simulink model "prob1"  (R2020b)
settings: Solver=VariableStepAuto  StartTime=0.0  StopTime=50.0  RelTol=1e-3
model workspace (MAT data in the model file):
  K1 = Simulink.Parameter
  K1.Value = 3
  K1.DataType = 'auto'
  K1.Dimensions = [1 1]
  K12 = Simulink.Parameter
  K12.Value = 3
  K12.DataType = 'auto'
  K12.Dimensions = [1 1]
  K12_M2 = 8
  b = Simulink.Parameter
  b.Value = 3
  b.DataType = 'auto'
  b.Dimensions = [1 1]
  k12 = Simulink.Parameter
  k12.Value = 3
  k12.DataType = 'auto'
  k12.Dimensions = [1 1]
  x1_M1 = 8
undefined symbols (not defined in the file): M1, M2
settings Model: OrderedModelArguments=off  Creator=HP  LastModifiedBy=HP

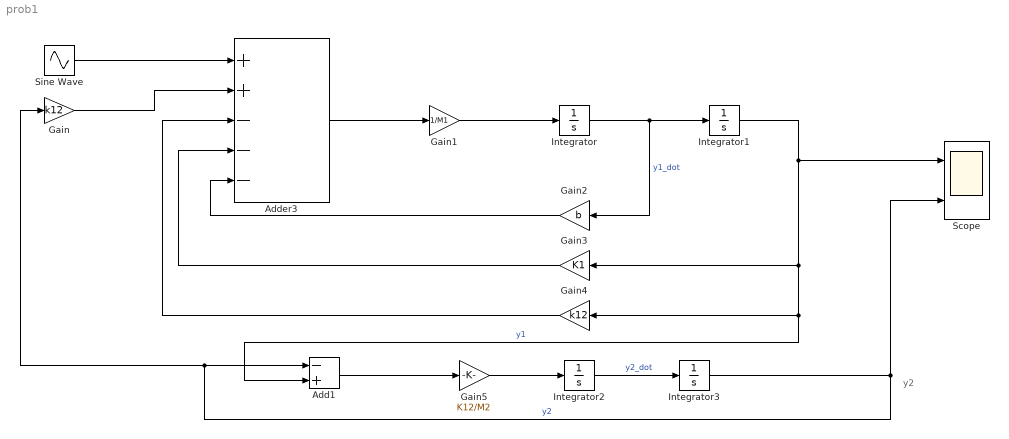
== system prob1 ==
  note: y2
  Add1 : Sum  Inputs=-+
  Adder3 : Sum  Inputs=++---
  Gain : Gain  Gain=k12
  Gain1 : Gain  Gain=1/M1
  Gain2 : Gain  Gain=b
  Gain3 : Gain  Gain=K1
  Gain4 : Gain  Gain=k12
  Gain5 : Gain  Gain=K12/M2
  Integrator{,1..3} (4 alike) : Integrator
  Scope : Scope  NumInputPorts=2
  Sine Wave : Sin  Amplitude=3  Frequency=10  SampleTime=0
  wires:
  Sine Wave/1 -> Adder3/1
  Gain/1 -> Adder3/2
  Adder3/1 -> Gain1/1
  Gain1/1 -> Integrator/1
  Integrator/1 -> Gain2/1, Integrator1/1  "y1_dot"
  Gain2/1 -> Adder3/5
  Gain3/1 -> Adder3/4
  Gain4/1 -> Adder3/3
  Add1/1 -> Gain5/1
  Gain5/1 -> Integrator2/1
  Integrator2/1 -> Integrator3/1  "y2_dot"
  Integrator1/1 -> Scope/1, Gain3/1, Gain4/1, Add1/2  "y1"
  Integrator3/1 -> Add1/1, Gain/1, Scope/2  "y2"
